simulink model "simulink_Feedback_con_y_sin_feedthrough_2017"  (R2017a)
settings: Solver=ode4  StartTime=0.0  StopTime=100  FixedStep=0.02  RelTol=1e-3
undefined symbols (not defined in the file or in its folder): Ad, Bd, Ld
libraries: dspstat3 x1
settings Model: Creator=PC  LastModifiedBy=q
settings DataIOCC: ReturnWorkspaceOutputs=on
settings SFSimCC: SimUseLocalCustomCode=on
settings RTWCC: RTWUseLocalCustomCode=on

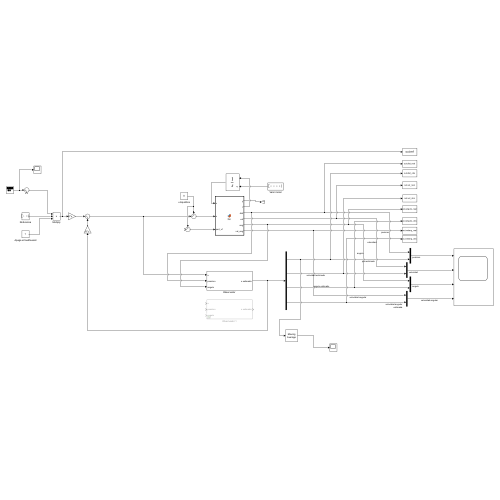
[thumbnail: Simulink's stored preview of the top-level diagram]
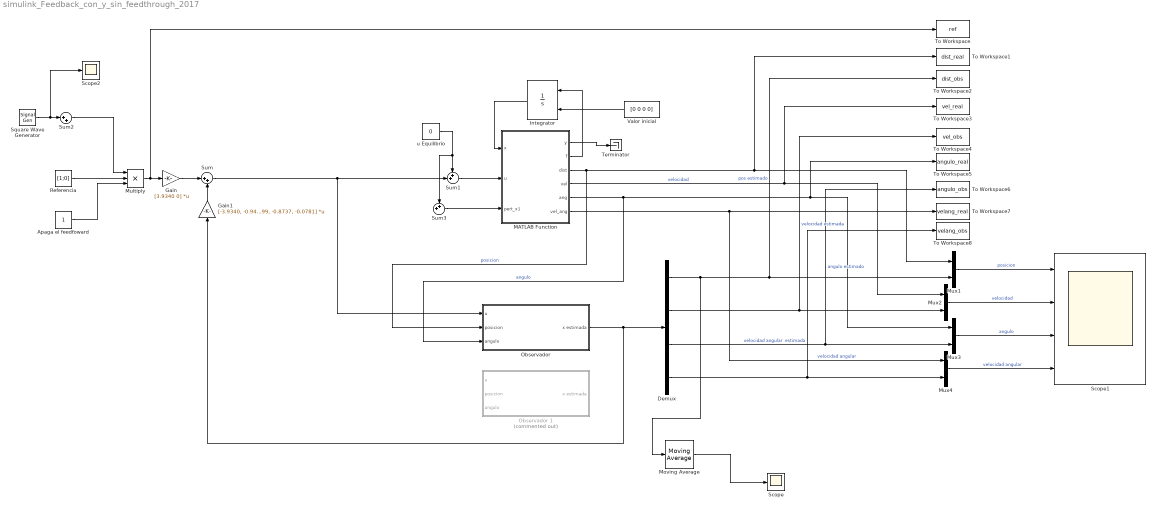
== system simulink_Feedback_con_y_sin_feedthrough_2017 ==
  Apaga el feedfoward : Constant
  Demux : Demux
  Gain : Gain  Gain=[3.9340 0]  Multiplication=Matrix(K*u)
  Gain1 : Gain  Gain=[-3.9340, -0.9499, -0.8737, -0.0781]  Multiplication=Matrix(K*u)
  Integrator : Integrator  InitialConditionSource=external
  MATLAB Function : MATLAB Function  TreatAsAtomicUnit=on
  Moving Average : dspstat3/Moving Average  Method=Sliding window  SpecifyWindowLength=on  WindowLength=5  ForgettingFactor=0.9  SimulateUsing=Code generation
  Multiply : Product  Inputs=3
  Mux{1..4} (4 alike) : Mux  Inputs=2
  "Observador " : Subsystem
  Observador 1 : Subsystem  Commented=on
  Referencia : Constant  Value=[1;0]
  Scope : Scope
  Scope1 : Scope  NumInputPorts=4
  Scope2 : Scope
  Square Wave Generator : SignalGenerator  WaveForm=square  Amplitude=-0.08  Frequency=0.125
  Sum : Sum  Inputs=|++
  Sum1 : Sum  Inputs=++|
  Sum2 : Sum  Inputs=|++
  Sum3 : Sum  Inputs=++|
  Terminator : Terminator
  To Workspace : ToWorkspace  VariableName=ref  SampleTime=0.02
  To Workspace1 : ToWorkspace  VariableName=dist_real  SampleTime=0.02
  To Workspace2 : ToWorkspace  VariableName=dist_obs  SampleTime=0.02
  To Workspace3 : ToWorkspace  VariableName=vel_real  SampleTime=0.02
  To Workspace4 : ToWorkspace  VariableName=vel_obs  SampleTime=0.02
  To Workspace5 : ToWorkspace  VariableName=angulo_real  SampleTime=0.02
  To Workspace6 : ToWorkspace  VariableName=angulo_obs  SampleTime=0.02
  To Workspace7 : ToWorkspace  VariableName=velang_real  SampleTime=0.02
  To Workspace8 : ToWorkspace  VariableName=velang_obs  SampleTime=0.02
  Valor inicial : Constant  Value=[0 0 0 0]
  u Equilibrio : Constant  Value=0
  wires:
  Valor inicial/1 -> Integrator/2
  MATLAB Function/2(f) -> Integrator/1
  u Equilibrio/1 -> Sum3/1, Sum1/1
  Sum1/1 -> MATLAB Function/2(u)
  Integrator/1 -> MATLAB Function/1(x)
  MATLAB Function/6(vel_ang) -> To Workspace7/1, Mux4/1  "velocidad angular"
  Demux/4 -> To Workspace8/1, Mux4/2  "velocidad angular  estimada"
  Mux1/1 -> Scope1/1  "posicion"
  Demux/1 -> Moving Average/1, Mux1/2, To Workspace2/1  "pos estimado"
  Mux2/1 -> Scope1/2  "velocidad"
  Mux4/1 -> Scope1/4  "velocidad angular"
  Demux/2 -> Mux2/2, To Workspace4/1  "velocidad estimada"
  Demux/3 -> To Workspace6/1, Mux3/2  "angulo estimado"
  MATLAB Function/5(ang) -> To Workspace5/1, Mux3/1, "Observador "/3(angulo)  "angulo"
  Mux3/1 -> Scope1/3  "angulo"
  MATLAB Function/4(vel) -> To Workspace3/1, Mux2/1  "velocidad"
  MATLAB Function/3(dist) -> "Observador "/2(posicion), To Workspace1/1, Mux1/1  "posicion"
  MATLAB Function/1(y) -> Terminator/1
  "Observador "/1(x estimada) -> Gain1/1, Demux/1
  Gain/1 -> Sum/1
  Gain1/1 -> Sum/2
  Sum/1 -> "Observador "/1(u), Sum1/2
  Multiply/1 -> To Workspace/1, Gain/1
  Referencia/1 -> Multiply/2
  Sum2/1 -> Multiply/1
  Apaga el feedfoward/1 -> Multiply/3
  Sum3/1 -> MATLAB Function/3(pert_x1)
  Moving Average/1 -> Scope/1
  Square Wave Generator/1 -> Scope2/1, Sum2/1

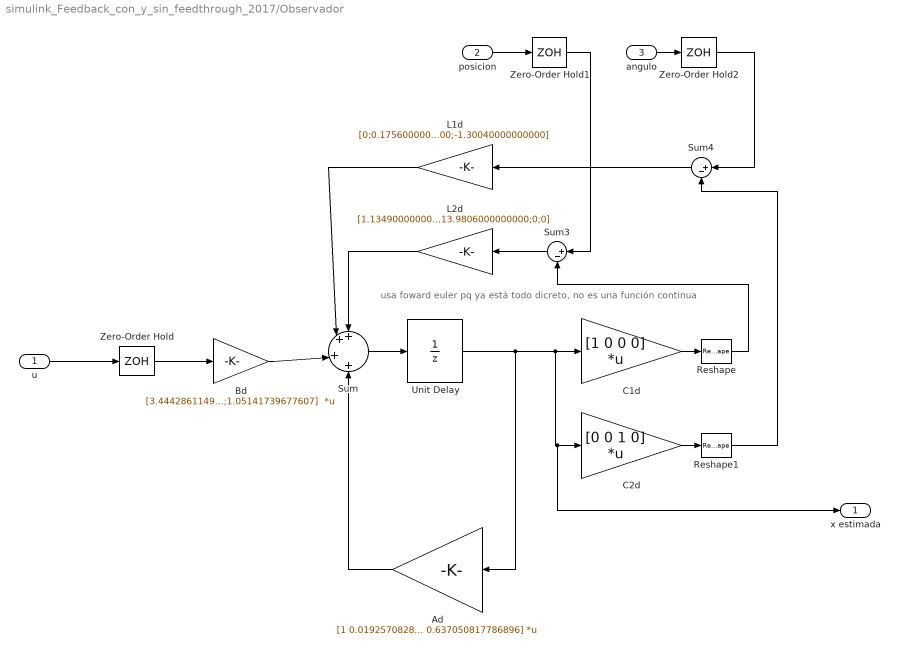
== system simulink_Feedback_con_y_sin_feedthrough_2017/Observador  ==
  note: usa foward euler pq ya está todo dicreto, no es una función continua
  u : Inport
  posicion : Inport  Port=2
  angulo : Inport  Port=3
  Ad : Gain  Gain=[1 0.0192570828996483 0.00170448697227250 1.03558375157804e-05;0 0.926639757552132 0.167521537510989 0.00148970690219522;0 0 0.973102548548734 0.0162030728429044;0 0 -2.50301828662619 0.637050817786896]  Multiplication=Matrix(K*u)
  Bd : Gain  Gain=[3.44428611496063e-06;0.000671990296398989;0.0112985384629050;1.05141739677607]  Multiplication=Matrix(K*u)
  C1d : Gain  Gain=[1 0 0 0]  Multiplication=Matrix(K*u)
  C2d : Gain  Gain=[0 0 1 0]  Multiplication=Matrix(K*u)
  L1d : Gain  Gain=[0;0.175600000000000;0.796300000000000;-1.30040000000000]
  L2d : Gain  Gain=[1.13490000000000;13.9806000000000;0;0]
  Reshape : Reshape
  Reshape1 : Reshape  OutputDimensions=[1]
  Sum : Sum  Inputs=++|+|+
  Sum3 : Sum  Inputs=|+-
  Sum4 : Sum  Inputs=|+-
  Unit Delay : UnitDelay  SampleTime=0.02  HasFrameUpgradeWarning=on
  Zero-Order Hold : ZeroOrderHold  SampleTime=0.02
  Zero-Order Hold1 : ZeroOrderHold  SampleTime=0.02
  Zero-Order Hold2 : ZeroOrderHold  SampleTime=0.02
  x estimada : Outport
  wires:
  Ad/1 -> Sum/4
  Sum/1 -> Unit Delay/1
  Bd/1 -> Sum/3
  Unit Delay/1 -> x estimada/1, C2d/1, C1d/1, Ad/1
  Sum4/1 -> L1d/1
  L2d/1 -> Sum/1
  C2d/1 -> Reshape1/1
  Reshape/1 -> Sum3/2
  Sum3/1 -> L2d/1
  L1d/1 -> Sum/2
  Reshape1/1 -> Sum4/2
  C1d/1 -> Reshape/1
  angulo/1 -> Zero-Order Hold2/1
  posicion/1 -> Zero-Order Hold1/1
  u/1 -> Zero-Order Hold/1
  Zero-Order Hold/1 -> Bd/1
  Zero-Order Hold1/1 -> Sum3/1
  Zero-Order Hold2/1 -> Sum4/1

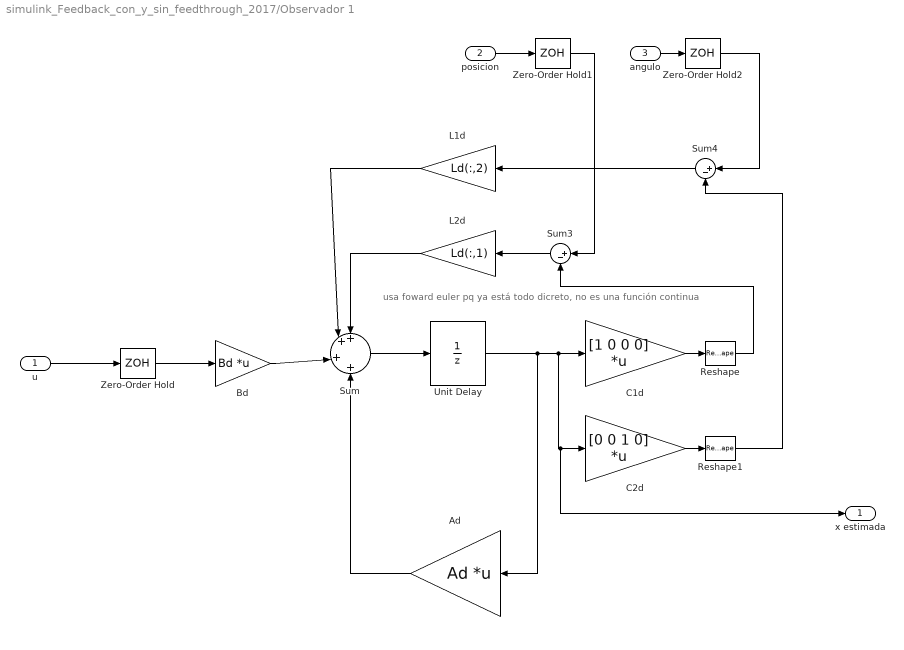
== system simulink_Feedback_con_y_sin_feedthrough_2017/Observador 1 ==
  note: usa foward euler pq ya está todo dicreto, no es una función continua
  u : Inport
  posicion : Inport  Port=2
  angulo : Inport  Port=3
  Ad : Gain  Gain=Ad  Multiplication=Matrix(K*u)
  Bd : Gain  Gain=Bd  Multiplication=Matrix(K*u)
  C1d : Gain  Gain=[1 0 0 0]  Multiplication=Matrix(K*u)
  C2d : Gain  Gain=[0 0 1 0]  Multiplication=Matrix(K*u)
  L1d : Gain  Gain=Ld(:,2)
  L2d : Gain  Gain=Ld(:,1)
  Reshape : Reshape
  Reshape1 : Reshape  OutputDimensions=[1]
  Sum : Sum  Inputs=++|+|+
  Sum3 : Sum  Inputs=|+-
  Sum4 : Sum  Inputs=|+-
  Unit Delay : UnitDelay  SampleTime=0.02  HasFrameUpgradeWarning=on
  Zero-Order Hold : ZeroOrderHold  SampleTime=0.02
  Zero-Order Hold1 : ZeroOrderHold  SampleTime=0.02
  Zero-Order Hold2 : ZeroOrderHold  SampleTime=0.02
  x estimada : Outport
  wires:
  Zero-Order Hold2/1 -> Sum4/1
  Zero-Order Hold1/1 -> Sum3/1
  Zero-Order Hold/1 -> Bd/1
  u/1 -> Zero-Order Hold/1
  posicion/1 -> Zero-Order Hold1/1
  angulo/1 -> Zero-Order Hold2/1
  C1d/1 -> Reshape/1
  Reshape1/1 -> Sum4/2
  L1d/1 -> Sum/2
  Sum3/1 -> L2d/1
  Reshape/1 -> Sum3/2
  C2d/1 -> Reshape1/1
  L2d/1 -> Sum/1
  Sum4/1 -> L1d/1
  Unit Delay/1 -> C1d/1, C2d/1, x estimada/1, Ad/1
  Bd/1 -> Sum/3
  Sum/1 -> Unit Delay/1
  Ad/1 -> Sum/4

== matlab function simulink_Feedback_con_y_sin_feedthrough_2017/MATLAB Function ==
  data: x input; u input; y output; f output; pert_x1 input; dist output; vel output; ang output; vel_ang output
function [y, f,dist,vel,ang,vel_ang] = fcn(x, u, pert_x1)
    
    g = 9.81; %kg m/s2
    m = 0.047; %kg
    kv = 0.2;
    R = 0.02;
    mr = 0.00275;
    J = 0.5*4*mr*power(R,2);
    
    x(1) = x(1) + pert_x1;

    %Dinamica
    f1 = x(2);
    f2 = (m*g*sin(x(3)) - kv * x(2)) * 1/(m + (J/power(R,2)));
    f3 = x(4);
    f4 = -20.73 * x(4) - 154.47*x(3) + u * 64.89;

    y = x(1);
    f = [f1 f2 f3 f4];
    dist=x(1);
    vel=x(2);
    ang=x(3);
    vel_ang=x(4);
end
